simulink model "magnetic_torque"  (R2020b)
settings: Solver=VariableStepAuto  StartTime=0.0  StopTime=10.0  RelTol=1e-3
undefined symbols (not defined in the file or in its folder): sim_constants
libraries: vrlib x1
settings Model: Creator=valerie  LastModifiedBy=valerie

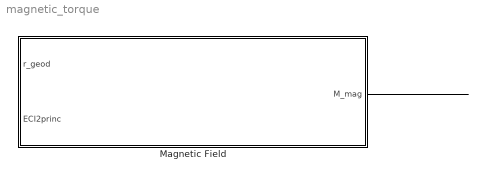
== system magnetic_torque ==
  Magnetic Field : Subsystem
  wires:
  ? -> Magnetic Field/2(ECI2princ)  "ECI2princ"
  ? -> Magnetic Field/1(r_geod)
  Magnetic Field/1(M_mag) -> ?

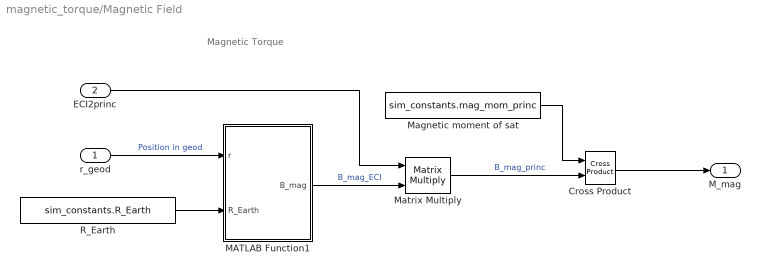
== system magnetic_torque/Magnetic Field ==
  note: Magnetic Torque
  r_geod : Inport
  ECI2princ : Inport  Port=2
  Cross Product : vrlib/Utilities/Cross Product
  MATLAB Function1 : MATLAB Function  TreatAsAtomicUnit=on
  Magnetic moment of sat : Constant  Value=sim_constants.mag_mom_princ
  Matrix Multiply : Product  Multiplication=Matrix(*)
  R_Earth : Constant  Value=sim_constants.R_Earth
  M_mag : Outport
  wires:
  r_geod/1 -> MATLAB Function1/1(r)  "Position in geod"
  Cross Product/1 -> M_mag/1
  MATLAB Function1/1(B_mag) -> Matrix Multiply/2  "B_mag_ECI"
  Magnetic moment of sat/1 -> Cross Product/1
  ECI2princ/1 -> Matrix Multiply/1
  Matrix Multiply/1 -> Cross Product/2  "B_mag_princ"
  R_Earth/1 -> MATLAB Function1/2(R_Earth)

== matlab function magnetic_torque/Magnetic Field/MATLAB Function1 ==
  data: r input; B_mag output; R_Earth input
function B_mag = magnetic_field(r, R_Earth)
% TODO: Fix me.
    B_mag = [0; 0; 0];
    
end
